simulink model "sampleModel1431"  (R2023a)
settings: Solver=VariableStepAuto  StartTime=0.0  StopTime=10.0  RelTol=1e-3
libraries: hdlsllib x3, simulink x1
settings Model: Creator=user1  LastModifiedBy=user1

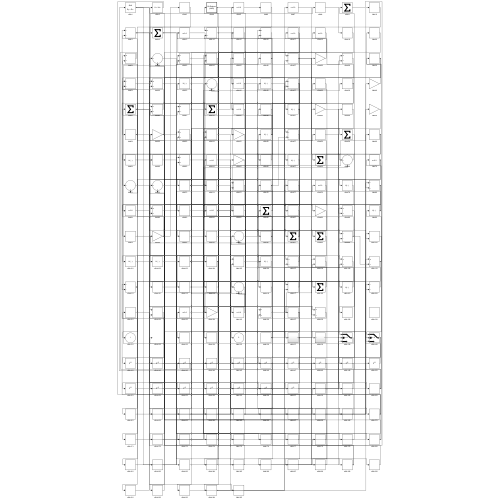
[thumbnail: Simulink's stored preview of the top-level diagram]
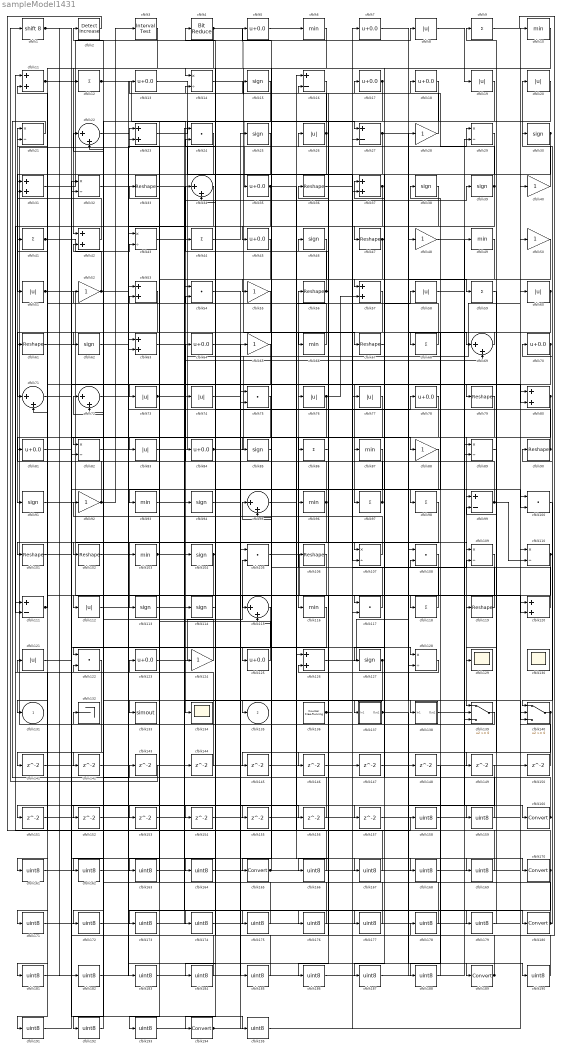
== system sampleModel1431 ==
  cfblk1 : ArithShift  BitShiftNumber=8
  cfblk{6,10,49,66,87,93,96,103,116} (9 alike) : MinMax
  cfblk{24,54,75,100,105,108,117,122} (8 alike) : DotProduct  OutDataTypeStr=Inherit: Inherit via internal rule
  cfblk{33,36,47,56,61,67,79,90,101..102,106,119} (12 alike) : Reshape
  cfblk{15,25,30,38..39,46,62,85,91,94,104,113..114,127} (14 alike) : Signum
  cfblk{14,21,29,32,43,82,89,107,109..110,128} (11 alike) : Product  Inputs=*/  RndMeth=Zero  SaturateOnIntegerOverflow=on
  cfblk{11,23,31,37,42,53,57,63,80,120,126} (11 alike) : Sum
  cfblk{16,27,99,111} (4 alike) : Sum  Inputs=+-
  cfblk{8,19..20,26,51,58,60,73..74,76..77,83,112,121} (14 alike) : Abs  SaturateOnIntegerOverflow=off
  cfblk{22,34,69,71..72,95,115} (7 alike) : Sum  Inputs=|++
  cfblk{9,12,41,44,59,68,86,97..98,118} (10 alike) : Sum  Inputs=+
  cfblk{5,7,13,17..18,35,45,64,70,78,81,84,123,125} (14 alike) : Bias  Bias=0.0  SaturateOnIntegerOverflow=off
  cfblk{28,40,48,50,52,55,65,88,92,124} (10 alike) : Gain
  cfblk129 : Scope
  cfblk130 : Scope
      settings: Floating=on
  cfblk132 : Terminator
  cfblk133 : ToWorkspace  VariableName=simout  SaveFormat=Timeseries  SampleTime=-1
  cfblk134 : Scope
  cfblk136 : hdlsllib/Sources/Counter Free-Running  NumBits=16  tsamp=-1
  cfblk137 : Subsystem
      settings: LibrarySourceBlock=|
      | hdlsllib/Ports &
      | Subsystems/Subsystem
  cfblk138 : Subsystem
      settings: LibrarySourceBlock=|
      | hdlsllib/Ports &
      | Subsystems/Subsystem
  cfblk139 : Switch  SaturateOnIntegerOverflow=off  InputSameDT=off
  cfblk140 : Switch  SaturateOnIntegerOverflow=off  InputSameDT=off
  cfblk{141..157} (17 alike) : Delay  SampleTime=1
  cfblk{158..159,161..164,166..169,171..179,181..188,190..193,195} (32 alike) : DataTypeConversion  OutDataTypeStr=uint8  SaturateOnIntegerOverflow=off  RndMeth=Floor
  cfblk{160,165,170,180,189,194} (6 alike) : DataTypeConversion  SaturateOnIntegerOverflow=off  RndMeth=Floor
  cfblk2 : simulink/Logic and Bit Operations/Detect Increase  vinit=0.0  OutDataTypeStr=boolean
      settings: LibrarySourceBlock=|
      | hdlsllib/Logic and Bit
      | Operations/Detect
      | Increase
  cfblk3 : hdlsllib/Logic and Bit Operations/Interval Test  IntervalClosedRight=on  uplimit=0.5  IntervalClosedLeft=on  lowlimit=-0.5  OutDataTypeStr=boolean
  cfblk4 : hdlsllib/Logic and Bit Operations/Bit Reduce  mode=AND
  cfblk131 : Outport  VectorParamsAs1DForOutWhenUnconnected=off
  cfblk135 : Outport  Port=2  VectorParamsAs1DForOutWhenUnconnected=off
  wires:
  cfblk140/1 -> cfblk145/1, cfblk146/1
  cfblk16/1 -> cfblk165/1
  cfblk77/1 -> cfblk83/1
  cfblk51/1 -> cfblk107/1, cfblk11/2
  cfblk90/1 -> cfblk82/1, cfblk14/2
  cfblk110/1 -> cfblk134/1, cfblk90/1
  cfblk68/1 -> cfblk14/1
  cfblk14/1 -> cfblk67/1
  cfblk139/1 -> cfblk23/1
  cfblk87/1 -> cfblk116/1
  cfblk117/1 -> cfblk56/1
  cfblk86/1 -> cfblk46/1
  cfblk6/1 -> cfblk135/1
  cfblk46/1 -> cfblk55/1
  cfblk91/1 -> cfblk117/1
  cfblk92/1 -> cfblk21/1, cfblk3/1
  cfblk18/1 -> cfblk133/1
  cfblk12/1 -> cfblk114/1, cfblk44/1
  cfblk83/1 -> cfblk29/1
  cfblk4/1 -> cfblk35/1, cfblk81/1
  cfblk37/1 -> cfblk47/1, cfblk95/2, cfblk61/1
  cfblk100/1 -> cfblk140/1
  cfblk119/1 -> cfblk5/1
  cfblk79/1 -> cfblk139/1
  cfblk80/1 -> cfblk96/1, cfblk125/1
  cfblk45/1 -> cfblk94/1
  cfblk118/1 -> cfblk37/1
  cfblk137/1(Out1) -> cfblk140/2, cfblk157/1, cfblk159/1
  cfblk128/1 -> cfblk126/2
  cfblk120/1 -> cfblk38/1
  cfblk25/1 -> cfblk51/1
  cfblk102/1 -> cfblk113/1
  cfblk32/1 -> cfblk189/1
  cfblk96/1 -> cfblk131/1, cfblk31/2
  cfblk44/1 -> cfblk25/1
  cfblk48/1 -> cfblk160/1
  cfblk66/1 -> cfblk41/1
  cfblk31/1 -> cfblk8/1
  cfblk138/1(Out1) -> cfblk29/2
  cfblk123/1 -> cfblk105/2
  cfblk28/1 -> cfblk15/1
  cfblk113/1 -> cfblk39/1
  cfblk27/1 -> cfblk45/1, cfblk140/3, cfblk69/1
  cfblk3/1 -> cfblk42/1
  cfblk99/1 -> cfblk64/1, cfblk110/2
  cfblk84/1 -> cfblk7/1, cfblk99/1
  cfblk98/1 -> cfblk101/1
  cfblk54/1 -> cfblk137/1(In1)
  cfblk53/1 -> cfblk122/1
  cfblk97/1 -> cfblk33/1, cfblk54/2
  cfblk114/1 -> cfblk84/1
  cfblk112/1 -> cfblk118/1
  cfblk23/1 -> cfblk27/1
  cfblk82/1 -> cfblk78/1
  cfblk55/1 -> cfblk71/1
  cfblk7/1 -> cfblk59/1
  cfblk107/1 -> cfblk92/1
  cfblk105/1 -> cfblk119/1
  cfblk61/1 -> cfblk97/1
  cfblk106/1 -> cfblk115/1
  cfblk125/1 -> cfblk53/2
  cfblk76/1 -> cfblk91/1, cfblk57/2
  cfblk71/1 -> cfblk88/1
  cfblk5/1 -> cfblk6/1
  cfblk93/1 -> cfblk120/2
  cfblk17/1 -> cfblk106/1, cfblk34/2
  cfblk59/1 -> cfblk129/1
  cfblk126/1 -> cfblk28/1
  cfblk73/1 -> cfblk40/1, cfblk69/2
  cfblk67/1 -> cfblk127/1
  cfblk19/1 -> cfblk104/1
  cfblk10/1 -> cfblk194/1
  cfblk38/1 -> cfblk111/2
  cfblk15/1 -> cfblk112/1
  cfblk30/1 -> cfblk82/2, cfblk73/1
  cfblk20/1 -> cfblk124/1
  cfblk39/1 -> cfblk66/1, cfblk18/1, cfblk155/1
  cfblk34/1 -> cfblk62/1
  cfblk95/1 -> cfblk58/1
  cfblk1/1 -> cfblk79/1, cfblk128/1, cfblk12/1
  cfblk56/1 -> cfblk34/1, cfblk36/1
  cfblk11/1 -> cfblk182/1, cfblk195/1
  cfblk85/1 -> cfblk115/2
  cfblk63/1 -> cfblk180/1
  cfblk60/1 -> cfblk85/1, cfblk98/1
  cfblk49/1 -> cfblk103/1
  cfblk127/1 -> cfblk152/1, cfblk163/1
  cfblk124/1 -> cfblk52/1
  cfblk42/1 -> cfblk31/1
  cfblk136/1 -> cfblk86/1, cfblk109/2
  cfblk36/1 -> cfblk109/1
  cfblk74/1 -> cfblk170/1
  cfblk70/1 -> cfblk71/2, cfblk89/2
  cfblk26/1 -> cfblk102/1, cfblk13/1
  cfblk13/1 -> cfblk107/2
  cfblk58/1 -> cfblk80/2
  cfblk8/1 -> cfblk19/1
  cfblk103/1 -> cfblk138/1(In1), cfblk128/2
  cfblk41/1 -> cfblk43/2, cfblk100/2
  cfblk40/1 -> cfblk20/1
  cfblk35/1 -> cfblk164/1, cfblk167/1
  cfblk47/1 -> cfblk87/1, cfblk93/1
  cfblk104/1 -> cfblk171/1, cfblk174/1
  cfblk29/1 -> cfblk57/1
  cfblk111/1 -> cfblk21/2, cfblk191/1
  cfblk69/1 -> cfblk68/1
  cfblk52/1 -> cfblk42/2, cfblk26/1
  cfblk57/1 -> cfblk141/1
  cfblk141/1 -> cfblk27/2
  cfblk116/1 -> cfblk142/1
  cfblk142/1 -> cfblk126/1
  cfblk21/1 -> cfblk143/1
  cfblk143/1 -> cfblk1/1
  cfblk144/1 -> cfblk111/1
  cfblk145/1 -> cfblk120/1
  cfblk89/1 -> cfblk149/1
  cfblk150/1 -> cfblk80/1
  cfblk122/1 -> cfblk151/1
  cfblk151/1 -> cfblk53/1
  cfblk152/1 -> cfblk139/2
  cfblk81/1 -> cfblk153/1
  cfblk153/1 -> cfblk23/2
  cfblk115/1 -> cfblk154/1
  cfblk154/1 -> cfblk117/2
  cfblk155/1 -> cfblk37/2
  cfblk101/1 -> cfblk156/1
  cfblk156/1 -> cfblk54/1
  cfblk157/1 -> cfblk139/3
  cfblk2/1 -> cfblk158/1
  cfblk158/1 -> cfblk60/1
  cfblk159/1 -> cfblk2/1
  cfblk160/1 -> cfblk30/1, cfblk99/2, cfblk17/1
  cfblk109/1 -> cfblk161/1
  cfblk161/1 -> cfblk48/1
  cfblk75/1 -> cfblk162/1
  cfblk162/1 -> cfblk144/1
  cfblk163/1 -> cfblk75/1
  cfblk164/1 -> cfblk75/2
  cfblk165/1 -> cfblk110/1, cfblk95/1, cfblk100/1
  cfblk146/1 -> cfblk166/1
  cfblk166/1 -> cfblk16/1
  cfblk167/1 -> cfblk16/2
  cfblk121/1 -> cfblk168/1
  cfblk168/1 -> cfblk50/1
  cfblk94/1 -> cfblk169/1
  cfblk169/1 -> cfblk121/1
  cfblk170/1 -> cfblk89/1, cfblk11/1, cfblk43/1, cfblk173/1
  cfblk171/1 -> cfblk74/1
  cfblk24/1 -> cfblk172/1
  cfblk172/1 -> cfblk150/1
  cfblk173/1 -> cfblk24/1
  cfblk174/1 -> cfblk24/2
  cfblk72/1 -> cfblk175/1
  cfblk175/1 -> cfblk105/1
  cfblk33/1 -> cfblk176/1
  cfblk176/1 -> cfblk72/1
  cfblk43/1 -> cfblk177/1
  cfblk177/1 -> cfblk72/2
  cfblk9/1 -> cfblk178/1
  cfblk178/1 -> cfblk123/1
  cfblk62/1 -> cfblk179/1
  cfblk179/1 -> cfblk9/1
  cfblk180/1 -> cfblk132/1, cfblk70/1
  cfblk149/1 -> cfblk181/1
  cfblk181/1 -> cfblk63/1
  cfblk182/1 -> cfblk63/2
  cfblk22/1 -> cfblk183/1
  cfblk183/1 -> cfblk148/1
  cfblk88/1 -> cfblk184/1
  cfblk184/1 -> cfblk22/1
  cfblk64/1 -> cfblk185/1
  cfblk185/1 -> cfblk22/2
  cfblk108/1 -> cfblk186/1
  cfblk186/1 -> cfblk49/1
  cfblk50/1 -> cfblk187/1
  cfblk187/1 -> cfblk108/1
  cfblk148/1 -> cfblk188/1
  cfblk188/1 -> cfblk108/2
  cfblk189/1 -> cfblk76/1, cfblk4/1
  cfblk147/1 -> cfblk190/1
  cfblk190/1 -> cfblk32/1
  cfblk191/1 -> cfblk32/2
  cfblk65/1 -> cfblk192/1
  cfblk192/1 -> cfblk122/2
  cfblk78/1 -> cfblk193/1
  cfblk193/1 -> cfblk65/1
  cfblk194/1 -> cfblk147/1, cfblk77/1
  cfblk195/1 -> cfblk10/1

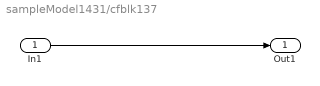
== system sampleModel1431/cfblk137 ==
  In1 : Inport
  Out1 : Outport
  wires:
  In1/1 -> Out1/1

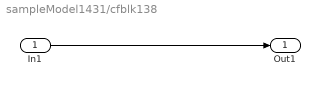
== system sampleModel1431/cfblk138 ==
  In1 : Inport
  Out1 : Outport
  wires:
  In1/1 -> Out1/1
